simulink model "IFSSIM_TireSuspension"  (R2025b)
settings: Solver=FixedStepDiscrete  StartTime=0  StopTime=inf  FixedStep=1/960  RelTol=1e-3
undefined symbols (not defined in the file): IFSSIM_WheelsBus_zero
settings Model: Creator=raulmoran  LastModifiedBy=raulmoran

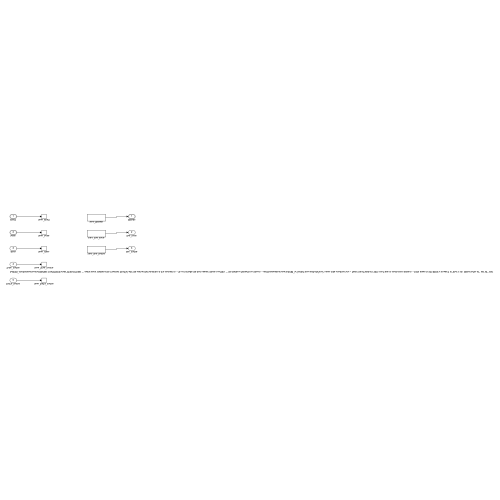
[thumbnail: Simulink's stored preview of the top-level diagram]
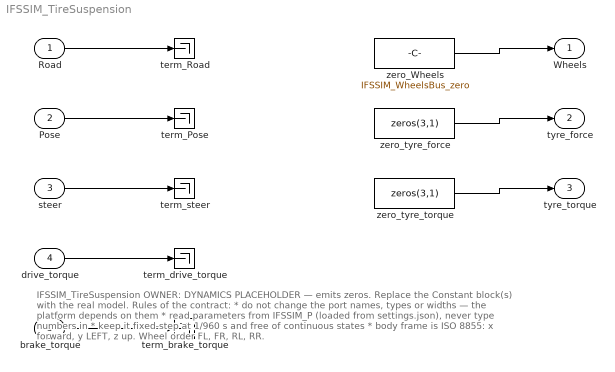
== system IFSSIM_TireSuspension ==
  note: IFSSIM_TireSuspension\n\nOWNER: DYNAMICS\n\nPLACEHOLDER — emits zeros. Replace the Constant block(s) with the real model.\n\nRules of the contract:\n * do not change the port names, types or widths — the platform depends on them\n * read parameters from IFSSIM_P (loaded from settings.json), never type numbers in\n * keep it fixed-step at 1/960 s and free of continuous states\n * body frame is ISO 8855: x forward, y LEFT, z up. Wheel order FL, FR, RL, RR.
  Road : Inport  OutDataTypeStr=Bus: IFSSIM_RoadBus  BusOutputAsStruct=on
  Pose : Inport  Port=2  OutDataTypeStr=Bus: IFSSIM_PoseBus  BusOutputAsStruct=on
  steer : Inport  Port=3  PortDimensions=4
  drive_torque : Inport  Port=4  PortDimensions=4
  brake_torque : Inport  Port=5  PortDimensions=4
  term_Pose : Terminator
  term_Road : Terminator
  term_brake_torque : Terminator
  term_drive_torque : Terminator
  term_steer : Terminator
  zero_Wheels : Constant  Value=IFSSIM_WheelsBus_zero  OutDataTypeStr=Bus: IFSSIM_WheelsBus
  zero_tyre_force : Constant  Value=zeros(3,1)
  zero_tyre_torque : Constant  Value=zeros(3,1)
  Wheels : Outport  OutDataTypeStr=Bus: IFSSIM_WheelsBus
  tyre_force : Outport  Port=2  PortDimensions=3
  tyre_torque : Outport  Port=3  PortDimensions=3
  wires:
  Road/1 -> term_Road/1
  Pose/1 -> term_Pose/1
  steer/1 -> term_steer/1
  drive_torque/1 -> term_drive_torque/1
  brake_torque/1 -> term_brake_torque/1
  zero_Wheels/1 -> Wheels/1
  zero_tyre_force/1 -> tyre_force/1
  zero_tyre_torque/1 -> tyre_torque/1
